simulink model "RollOnlySimulation"  (R2012b)
settings: Solver=ode45  StartTime=0.0  StopTime=10  RelTol=1e-3
values from neighbouring files (symbols this model uses):
  A_matrix = veh.StateToStateRates    [InitSimuLinkModel_basic00.m]
  B_matrix = [0; veh.Ixx]    [InitSimuLinkModel_basic00.m]
  Q_matrix = [0.01 0; 0 0.01]    [InitSimuLinkModel_basic00.m]
  R_matrix = [0.1 0 0; 0 0.1 0; 0 0 .001]    [InitSimuLinkModel_basic00.m]
undefined symbols (not defined in the file or in its folder): cont, env, inp, sen, sigbuilder_block
settings Model: Creator=admin  LastModifiedBy=admin

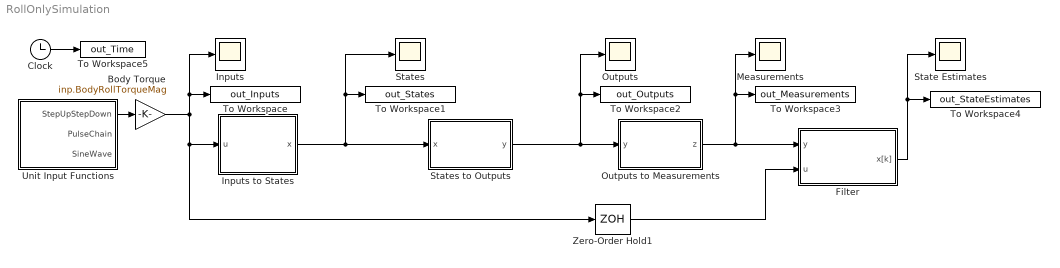
== system RollOnlySimulation ==
  Body Torque : Gain  Gain=inp.BodyRollTorqueMag
  Clock : Clock
  Filter : Subsystem
  Inputs : Scope
      settings: TimeRange=10  YMin=-10  YMax=10
  Inputs to States : Subsystem
  Measurements : Scope
      settings: TimeRange=10  YMin=-2  YMax=10  SaveName=ScopeData4
  Outputs : Scope
      settings: TimeRange=10  YMin=-2  YMax=10  SaveName=ScopeData2
  Outputs to Measurements : Subsystem
  State Estimates : Scope
      settings: TimeRange=10  YMin=-0.8  YMax=0.6000000000000001  SaveName=ScopeData3
  States : Scope
      settings: TimeRange=10  YMin=-0.5  YMax=0.5
  States to Outputs : Subsystem
  To Workspace : ToWorkspace  VariableName=out_Inputs  SampleTime=cont.LoopPeriod
  To Workspace1 : ToWorkspace  VariableName=out_States  SampleTime=cont.LoopPeriod
  To Workspace2 : ToWorkspace  VariableName=out_Outputs  SampleTime=cont.LoopPeriod
  To Workspace3 : ToWorkspace  VariableName=out_Measurements  SampleTime=-1
  To Workspace4 : ToWorkspace  VariableName=out_StateEstimates  SampleTime=-1
  To Workspace5 : ToWorkspace  VariableName=out_Time  SampleTime=cont.LoopPeriod
  Unit Input Functions : Subsystem
  Zero-Order Hold1 : ZeroOrderHold  SampleTime=cont.LoopPeriod
  wires:
  Unit Input Functions/1(StepUpStepDown) -> Body Torque/1
  Body Torque/1 -> Inputs to States/1(u), Zero-Order Hold1/1, To Workspace/1, Inputs/1
  Filter/1(x[k]) -> To Workspace4/1, State Estimates/1
  Zero-Order Hold1/1 -> Filter/2(u)
  States to Outputs/1(y) -> To Workspace2/1, Outputs/1, Outputs to Measurements/1(y)
  Inputs to States/1(x) -> To Workspace1/1, States/1, States to Outputs/1(x)
  Outputs to Measurements/1(z) -> To Workspace3/1, Measurements/1, Filter/1(y)
  Clock/1 -> To Workspace5/1

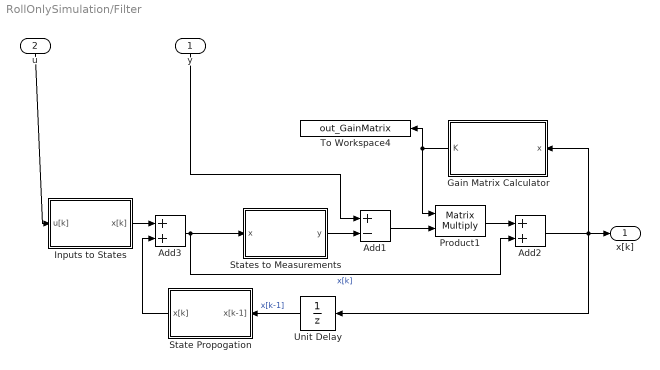
== system RollOnlySimulation/Filter ==
  y : Inport
  u : Inport  Port=2
  Add1 : Sum  Inputs=+-  SampleTime=cont.LoopPeriod
  Add2 : Sum  SampleTime=cont.LoopPeriod
  Add3 : Sum  SampleTime=cont.LoopPeriod
  Gain Matrix Calculator : Subsystem
  Inputs to States : Subsystem
  Product1 : Product  Multiplication=Matrix(*)  RndMeth=Zero
  State Propogation : Subsystem
  States to Measurements : Subsystem
  To Workspace4 : ToWorkspace  VariableName=out_GainMatrix  SampleTime=-1
  Unit Delay : UnitDelay  InitialCondition=[0; 0]  SampleTime=cont.LoopPeriod
  x[k] : Outport
  wires:
  Add3/1 -> States to Measurements/1(x), Add2/2  "x[k]"
  Unit Delay/1 -> State Propogation/1(x[k-1])  "x[k-1]"
  Product1/1 -> Add2/1
  y/1 -> Add1/1
  Add1/1 -> Product1/2
  Add2/1 -> x[k]/1, Gain Matrix Calculator/1(x), Unit Delay/1
  States to Measurements/1(y) -> Add1/2
  Gain Matrix Calculator/1(K) -> Product1/1, To Workspace4/1
  u/1 -> Inputs to States/1(u[k])
  Inputs to States/1(x[k]) -> Add3/1
  State Propogation/1(x[k]) -> Add3/2

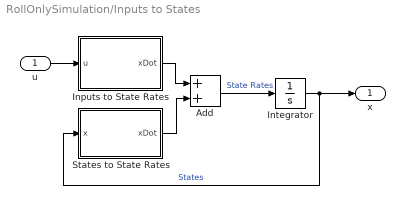
== system RollOnlySimulation/Inputs to States ==
  u : Inport
  Add : Sum
  Inputs to State Rates : Subsystem
  Integrator : Integrator  InitialCondition=[0; 0]
  States to State Rates : Subsystem
  x : Outport
  wires:
  States to State Rates/1(xDot) -> Add/2
  u/1 -> Inputs to State Rates/1(u)
  Inputs to State Rates/1(xDot) -> Add/1
  Add/1 -> Integrator/1  "State Rates"
  Integrator/1 -> x/1, States to State Rates/1(x)  "States"

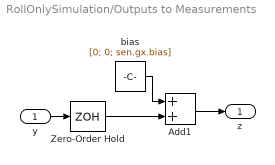
== system RollOnlySimulation/Outputs to Measurements ==
  y : Inport
  Add1 : Sum
  Zero-Order Hold : ZeroOrderHold  SampleTime=cont.LoopPeriod
  bias : Constant  Value=[0; 0; sen.gx.bias]  SampleTime=cont.LoopPeriod
  z : Outport
  wires:
  Zero-Order Hold/1 -> Add1/2
  bias/1 -> Add1/1
  Add1/1 -> z/1
  y/1 -> Zero-Order Hold/1

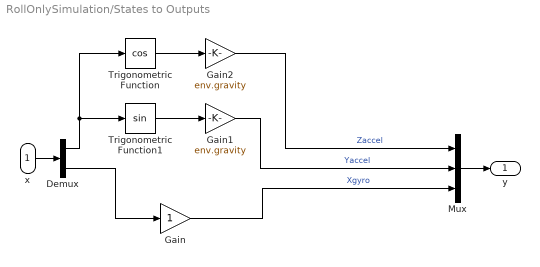
== system RollOnlySimulation/States to Outputs ==
  x : Inport
  Demux : Demux  Outputs=2
  Gain : Gain
  Gain1 : Gain  Gain=env.gravity
  Gain2 : Gain  Gain=env.gravity
  Mux : Mux  Inputs=3
  Trigonometric Function : Trigonometry  Operator=cos
  Trigonometric Function1 : Trigonometry
  y : Outport
  wires:
  x/1 -> Demux/1
  Demux/2 -> Gain/1
  Demux/1 -> Trigonometric Function1/1, Trigonometric Function/1
  Trigonometric Function1/1 -> Gain1/1
  Trigonometric Function/1 -> Gain2/1
  Mux/1 -> y/1
  Gain2/1 -> Mux/1  "Zaccel"
  Gain1/1 -> Mux/2  "Yaccel"
  Gain/1 -> Mux/3  "Xgyro"

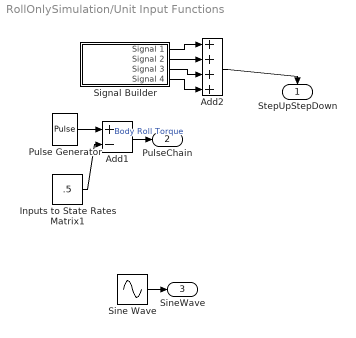
== system RollOnlySimulation/Unit Input Functions ==
  Add1 : Sum  Inputs=+-
  Add2 : Sum  Inputs=++++
  Inputs to State Rates Matrix1 : Constant  Value=.5  SampleTime=cont.LoopPeriod
  Pulse Generator : DiscretePulseGenerator  PulseType=Time based  Period=10  PulseWidth=50
  Signal Builder : Subsystem  Tag=STV Subsys  LoadFcn=sigbuilder_block('load');  StartFcn=sigbuilder_block('start');  StopFcn=sigbuilder_block('stop');  ClipboardFcn=sigbuilder_block('clipboard');  mask(Sigbuilder block){}
      mask help: Simulink:masks:SigbuilderBlock_MD
      mask init:
      | if ~strcmp(get_param(bdroot(gcbh),'SimulationStatus'),'stopped') tuvar = sigbuilder_block('maskInit'); end
      settings: CopyFcn=sigbuilder_block('copy');  DeleteFcn=sigbuilder_block('delete');  ModelCloseFcn=sigbuilder_block('modelClose');  PreSaveFcn=sigbuilder_block('preSave');  PauseFcn=sigbuilder_block('pause');  ContinueFcn=sigbuilder_block('continue');  NameChangeFcn=sigbuilder_block('namechange');  OpenFcn=sigbuilder_block('open',[406.5 147 550.5 399.75 ]);  CloseFcn=sigbuilder_block('close');
      mask Display: plot(0, 0, 100, 100,[2, 2, 32, 32, 2], [68, 8, 8, 68, 68],[32, 2], [38, 38], [32, 19, 2],[53, 60, 44], [32, 17, 17, 2],[16, 16, 31, 31]);txt = getActiveGroup(gcbh);text(2, 100, txt,'verticalAlignment', 'top');
  Sine Wave : Sin  SampleTime=0
  StepUpStepDown : Outport
  PulseChain : Outport  Port=2
  SineWave : Outport  Port=3
  wires:
  Pulse Generator/1 -> Add1/1
  Inputs to State Rates Matrix1/1 -> Add1/2
  Signal Builder/1(Signal 1) -> Add2/1
  Add2/1 -> StepUpStepDown/1
  Sine Wave/1 -> SineWave/1
  Signal Builder/4(Signal 4) -> Add2/4
  Signal Builder/2(Signal 2) -> Add2/2
  Signal Builder/3(Signal 3) -> Add2/3
  Add1/1 -> PulseChain/1  "Body Roll Torque"

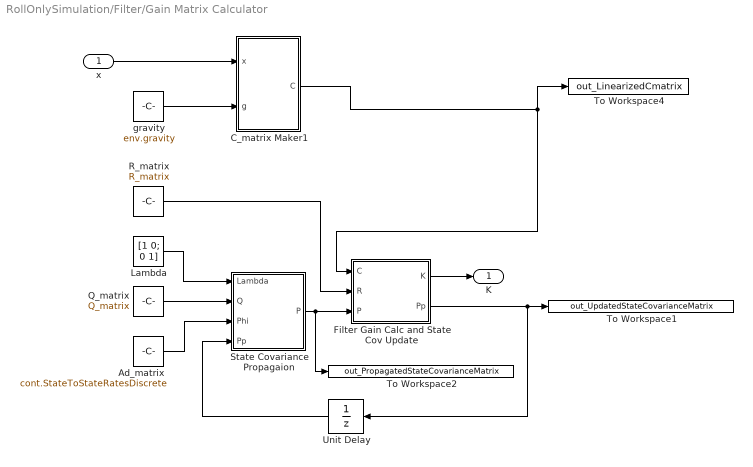
== system RollOnlySimulation/Filter/Gain Matrix Calculator ==
  x : Inport
  Ad_matrix : Constant  Value=cont.StateToStateRatesDiscrete  SampleTime=cont.LoopPeriod
  C_matrix Maker1 : MATLAB Function  TreatAsAtomicUnit=on
  Filter Gain Calc and State Cov Update : Subsystem
  Lambda : Constant  Value=[1 0; 0 1]  SampleTime=cont.LoopPeriod
  Q_matrix : Constant  Value=Q_matrix  SampleTime=cont.LoopPeriod
  R_matrix : Constant  Value=R_matrix  SampleTime=cont.LoopPeriod
  State Covariance Propagaion : MATLAB Function  TreatAsAtomicUnit=on
  To Workspace1 : ToWorkspace  VariableName=out_UpdatedStateCovarianceMatrix  SampleTime=-1
  To Workspace2 : ToWorkspace  VariableName=out_PropagatedStateCovarianceMatrix  SampleTime=-1
  To Workspace4 : ToWorkspace  VariableName=out_LinearizedCmatrix  SampleTime=-1
  Unit Delay : UnitDelay  InitialCondition=[0.001 0; 0 0.001]  SampleTime=cont.LoopPeriod
  gravity : Constant  Value=env.gravity  SampleTime=cont.LoopPeriod
  K : Outport
  wires:
  Unit Delay/1 -> State Covariance Propagaion/4(Pp)
  Q_matrix/1 -> State Covariance Propagaion/2(Q)
  Lambda/1 -> State Covariance Propagaion/1(Lambda)
  Ad_matrix/1 -> State Covariance Propagaion/3(Phi)
  R_matrix/1 -> Filter Gain Calc and State Cov Update/2(R)
  State Covariance Propagaion/1(P) -> To Workspace2/1, Filter Gain Calc and State Cov Update/3(P)
  Filter Gain Calc and State Cov Update/1(K) -> K/1
  Filter Gain Calc and State Cov Update/2(Pp) -> To Workspace1/1, Unit Delay/1
  C_matrix Maker1/1(C) -> To Workspace4/1, Filter Gain Calc and State Cov Update/1(C)
  x/1 -> C_matrix Maker1/1(x)
  gravity/1 -> C_matrix Maker1/2(g)

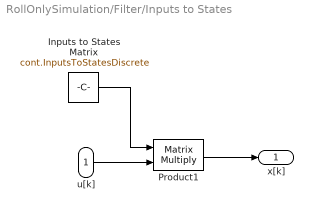
== system RollOnlySimulation/Filter/Inputs to States ==
  u[k] : Inport
  Inputs to States Matrix : Constant  Value=cont.InputsToStatesDiscrete  SampleTime=cont.LoopPeriod
  Product1 : Product  Multiplication=Matrix(*)  RndMeth=Zero
  x[k] : Outport
  wires:
  u[k]/1 -> Product1/2
  Inputs to States Matrix/1 -> Product1/1
  Product1/1 -> x[k]/1

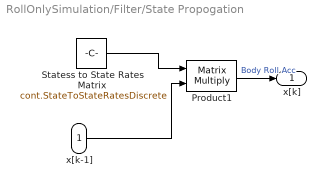
== system RollOnlySimulation/Filter/State Propogation ==
  x[k-1] : Inport
  Product1 : Product  Multiplication=Matrix(*)  RndMeth=Zero
  Statess to State Rates Matrix : Constant  Value=cont.StateToStateRatesDiscrete  SampleTime=cont.LoopPeriod
  x[k] : Outport
  wires:
  Product1/1 -> x[k]/1  "Body Roll Acc"
  x[k-1]/1 -> Product1/2
  Statess to State Rates Matrix/1 -> Product1/1

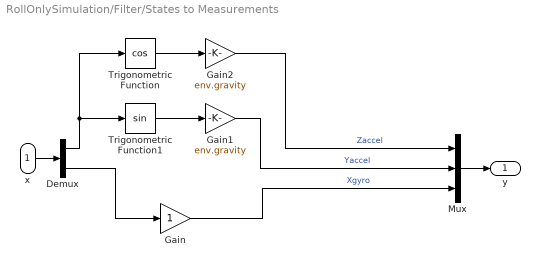
== system RollOnlySimulation/Filter/States to Measurements ==
  x : Inport
  Demux : Demux  Outputs=2
  Gain : Gain
  Gain1 : Gain  Gain=env.gravity
  Gain2 : Gain  Gain=env.gravity
  Mux : Mux  Inputs=3
  Trigonometric Function : Trigonometry  Operator=cos
  Trigonometric Function1 : Trigonometry
  y : Outport
  wires:
  x/1 -> Demux/1
  Demux/2 -> Gain/1
  Demux/1 -> Trigonometric Function1/1, Trigonometric Function/1
  Trigonometric Function1/1 -> Gain1/1
  Trigonometric Function/1 -> Gain2/1
  Mux/1 -> y/1
  Gain2/1 -> Mux/1  "Zaccel"
  Gain1/1 -> Mux/2  "Yaccel"
  Gain/1 -> Mux/3  "Xgyro"

== system RollOnlySimulation/Inputs to States/Inputs to State Rates ==
  u : Inport
  Inputs to State Rates Matrix : Constant  Value=B_matrix
  Product : Product  Multiplication=Matrix(*)  RndMeth=Zero
  xDot : Outport
  wires:
  u/1 -> Product/2
  Product/1 -> xDot/1
  Inputs to State Rates Matrix/1 -> Product/1

== system RollOnlySimulation/Inputs to States/States to State Rates ==
  x : Inport
  Product1 : Product  Multiplication=Matrix(*)  RndMeth=Zero
  Statess to State Rates Matrix : Constant  Value=A_matrix
  xDot : Outport
  wires:
  Product1/1 -> xDot/1  "Body Roll Acc"
  x/1 -> Product1/2
  Statess to State Rates Matrix/1 -> Product1/1

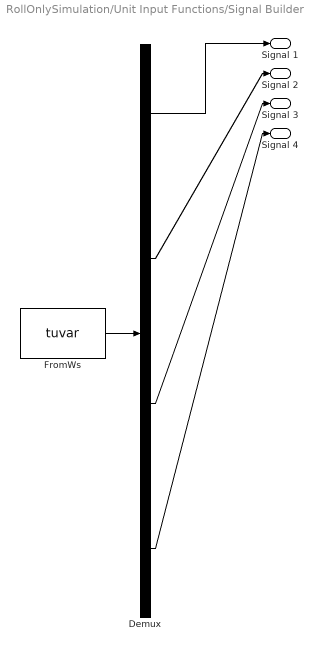
== system RollOnlySimulation/Unit Input Functions/Signal Builder ==
  Demux : Demux  Tag=STV Demux
  FromWs : FromWorkspace  Tag=STV FromWs  VariableName=tuvar  SampleTime=0
      SigBuilderData=|
      | common.afterFinalStr = 'Extrapolate'
      | common.sampleTime = 0
      | dataSet.timeRange = [0 10]
      | dataSet.name = 'Group 1'
      | sbobj.Groups.Name = 'Group 1'
      | sbobj.Groups.Signals(1).Name = 'Signal 1'
      | sbobj.Groups.Signals(1).XData = [0 1 1 2 2 10]
      | sbobj.Groups.Signals(1).YData = [0 0 1 1 0 0]
      | sbobj.Groups.Signals(2).Name = 'Signal 2'
      | sbobj.Groups.Signals(2).XData = [0 2 2 3 3 10]
      | sbobj.Groups.Signals(2).YData = [0 0 -1 -1 0 0]
      | sbobj.Groups.Signals(3).Name = 'Signal 3'
      | sbobj.Groups.Signals(3).XData = [0 4 4 5 5 10]
      | sbobj.Groups.Signals(3).YData = [0 0 -1 -1 0 0]
      | sbobj.Groups.Signals(4).Name = 'Signal 4'
      | sbobj.Groups.Signals(4).XData = [0 5 5 6 6 10]
      | sbobj.Groups.Signals(4).YData = [0 0 1 1 0 0]
  Signal 1 : Outport  Tag=STV Outport
  Signal 2 : Outport  Tag=STV Outport  Port=2
  Signal 3 : Outport  Tag=STV Outport  Port=3
  Signal 4 : Outport  Tag=STV Outport  Port=4
  wires:
  Demux/1 -> Signal 1/1
  FromWs/1 -> Demux/1
  Demux/2 -> Signal 2/1
  Demux/3 -> Signal 3/1
  Demux/4 -> Signal 4/1

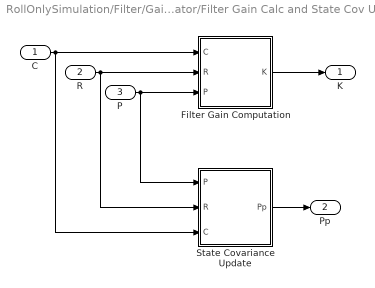
== system RollOnlySimulation/Filter/Gain Matrix Calculator/Filter Gain Calc and State Cov Update ==
  C : Inport  PortDimensions=[3 2]
  R : Inport  Port=2
  P : Inport  Port=3
  Filter Gain Computation : MATLAB Function  TreatAsAtomicUnit=on
  State Covariance Update : MATLAB Function  TreatAsAtomicUnit=on
  K : Outport
  Pp : Outport  Port=2
  wires:
  C/1 -> Filter Gain Computation/1(C), State Covariance Update/3(C)
  R/1 -> State Covariance Update/2(R), Filter Gain Computation/2(R)
  State Covariance Update/1(Pp) -> Pp/1
  P/1 -> State Covariance Update/1(P), Filter Gain Computation/3(P)
  Filter Gain Computation/1(K) -> K/1

== matlab function RollOnlySimulation/Filter/Gain Matrix Calculator/State Covariance Propagaion ==
  data: Lambda input; Q input; Phi input; P output; Pp input
function P = fcn(Lambda, Q, Phi,  Pp)
%#codegen

P=Phi*Pp*Phi' + Lambda*Q*Lambda';

== matlab function RollOnlySimulation/Filter/Gain Matrix Calculator/Filter Gain Calc and State Cov Update/Filter Gain Computation ==
  data: C input; R input; P input; K output
function K = fcn(C, R, P)
%#codegen

K=P*C'*(C*P*C'+R)^-1;

== matlab function RollOnlySimulation/Filter/Gain Matrix Calculator/Filter Gain Calc and State Cov Update/State Covariance Update ==
  data: P input; R input; Pp output; C input
function Pp = fcn(P, R, C)
%#codegen

Pp=(P^-1+C'*R^-1*C)^-1;

== matlab function RollOnlySimulation/Filter/Gain Matrix Calculator/C_matrix Maker1 ==
  data: x input; C output; g input
function C = fcn(x, g)
%#codegen

C = [-g*sin(x(1)), 0; g*cos(x(1)), 0; 0, 1];
